simulink model "LFPrzeszkoda"  (R2024a)
settings: Solver=FixedStepDiscrete  StartTime=0.0  StopTime=2500  FixedStep=0.01  RelTol=1e-3
undefined symbols (not defined in the file): DiscIntNeverNeededParam, lineLength, mapForSim
libraries: mobileRoboticsTrainingLib x3, slpidlib x2
settings Model: PacingRate=50  Creator=KMPKM  LastModifiedBy=Pawel
settings RTWCC: GPUComputeCapability=3.5

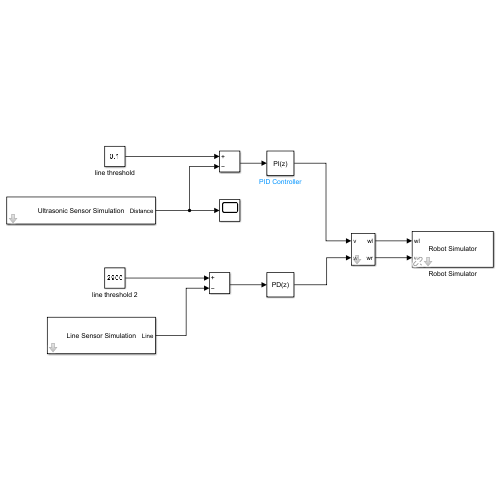
[thumbnail: Simulink's stored preview of the top-level diagram]
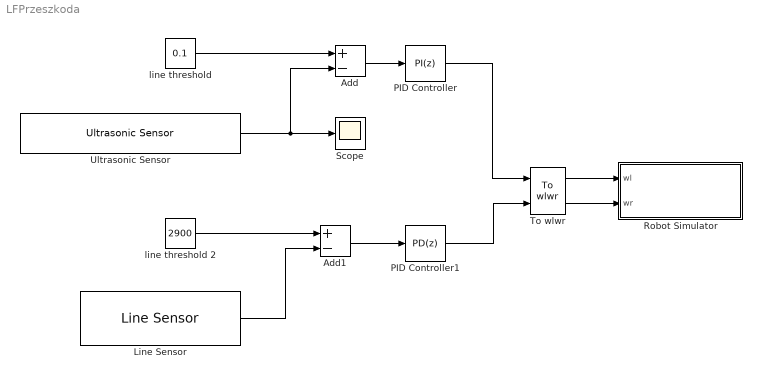
== system LFPrzeszkoda ==
  Add : Sum  Inputs=+-
  Add1 : Sum  Inputs=+-
  Line Sensor : mobileRoboticsTrainingLib/Line Sensor  mapVariable=mapForSim  envVal=2850  lineVal=2950  sensOff=[0.01 0]
      settings: SourceProductName=Mobile Robotics Training Library
  PID Controller : slpidlib/PID Controller  Controller=PI  Form=Parallel  TimeDomain=Discrete-time  UseExternalTs=off  SampleTime=-1  IntegratorMethod=Forward Euler  FilterMethod=Forward Euler  ControllerParametersSource=internal  P=1  I=0.001  UseKiTs=off  D=0.001  UseExternalDerivativeSource=off  N=100  UseFilter=on  TunerSelectOption=Transfer Function Based (PID Tuner App)  InitialConditionSource=internal  InitialConditionForIntegrator=0  InitialConditionForFilter=0  DifferentiatorICPrevScaledInput=0  ExternalReset=none  TrackingMode=off  Kt=1  LimitOutput=off  SatLimitsSource=internal  UpperSaturationLimit=inf  LowerSaturationLimit=-inf  LinearizeAsGain=on  AntiWindupMode=none  Kb=1  LimitIntegrator=off  UpperIntegratorSaturationLimit=inf  LowerIntegratorSaturationLimit=-inf  POutMin=[]  POutMax=[]  IOutMin=[]  IOutMax=[]  DOutMin=[]  DOutMax=[]  NOutMin=[]  NOutMax=[]  SumOutMin=[]  SumOutMax=[]  SaturationOutMin=[]  SaturationOutMax=[]  PParamMin=[]  PParamMax=[]  IParamMin=[]  IParamMax=[]  DParamMin=[]  DParamMax=[]  NParamMin=[]  NParamMax=[]  KbParamMin=[]  KbParamMax=[]  KtParamMin=[]  KtParamMax=[]  KbOutMin=[]  KbOutMax=[]  KtOutMin=[]  KtOutMax=[]  IntegratorOutMin=[]  IntegratorOutMax=[]  FilterOutMin=[]  FilterOutMax=[]  SumI1OutMin=[]  SumI1OutMax=[]  SumI2OutMin=[]  SumI2OutMax=[]  SumI3OutMin=[]  SumI3OutMax=[]  SumI4OutMin=[]  SumI4OutMax=[]  SumDOutMin=[]  SumDOutMax=[]  DifferentiatorOutMin=[]  DifferentiatorOutMax=[]  FilterDiffOutCoefMin=[]  FilterDiffOutCoefMax=[]  ReciprocalOutMin=[]  ReciprocalOutMax=[]  SumDenOutMin=[]  SumDenOutMax=[]  SumNumOutMin=[]  SumNumOutMax=[]  DivideOutMin=[]  DivideOutMax=[]  UdiffTsProdOutMin=[]  UdiffTsProdOutMax=[]  NTsProdOutMin=[]  NTsProdOutMax=[]  UintegralTsProdOutMin=[]  UintegralTsProdOutMax=[]  UngainTsProdOutMin=[]  UngainTsProdOutMax=[]  ClampingZeroOutDataTypeStr=Inherit: Inherit via back propagation  ClampingZeroOutMin=[]  ClampingZeroOutMax=[]  FilterDenConstantOutDataTypeStr=Inherit: Inherit via back propagation  FilterDenConstantOutMin=[]  FilterDenConstantOutMax=[]  PCopyOutDataTypeStr=Inherit: Inherit via back propagation  PCopyOutMin=[]  PCopyOutMax=[]  NCopyOutDataTypeStr=Inherit: Inherit via back propagation  NCopyOutMin=[]  NCopyOutMax=[]  IntegratorContinuousStateAttributes=''  IntegratorStateMustResolveToSignalObject=off  IntegratorRTWStateStorageClass=Auto  FilterContinuousStateAttributes=''  FilterStateMustResolveToSignalObject=off  FilterRTWStateStorageClass=Auto  ParallelPVariant=InternalParameters  IdealPVariant=Disabled  IVariant=InternalParameters  DVariant=Disabled  IntegratorVariant=Discrete  SatVariant=Disabled  AWVariant=Passthrough  PCopyVariant=Disabled  TRVariant=Disabled  FdbkBlocksVariant=Forward  IdealPFdbkVariant=Disabled  SatFdbkVariant=Disabled  DerivativeFilterVariant=Disabled  NVariant=Disabled  NCopyVariant=Disabled_SignalSpec  FilterICVariant=Disabled  IntegratorICVariant=InternalICs  ExternalResetVariant=Disabled  TRSumVariant=Passthrough  SumFdbkVariant=Disabled  SumVariant=Sum_PI  TsampFilterVariant=InternalTs  TsampNgainVariant=Passthrough  TsampIntegralVariant=Disabled_SignalSpec  ExternalSaturationOutDataTypeStr=Inherit: Same as second input  DerivativeSourceVariant=Disabled
  PID Controller1 : slpidlib/PID Controller  Controller=PD  Form=Parallel  TimeDomain=Discrete-time  UseExternalTs=off  SampleTime=-1  IntegratorMethod=Forward Euler  FilterMethod=Forward Euler  ControllerParametersSource=internal  P=0.01  I=1  UseKiTs=off  D=0.001  UseExternalDerivativeSource=off  N=100  UseFilter=on  TunerSelectOption=Transfer Function Based (PID Tuner App)  InitialConditionSource=internal  InitialConditionForIntegrator=0  InitialConditionForFilter=0  DifferentiatorICPrevScaledInput=0  ExternalReset=none  TrackingMode=off  Kt=1  LimitOutput=off  SatLimitsSource=internal  UpperSaturationLimit=inf  LowerSaturationLimit=-inf  LinearizeAsGain=on  AntiWindupMode=none  Kb=1  LimitIntegrator=off  UpperIntegratorSaturationLimit=inf  LowerIntegratorSaturationLimit=-inf  POutMin=[]  POutMax=[]  IOutMin=[]  IOutMax=[]  DOutMin=[]  DOutMax=[]  NOutMin=[]  NOutMax=[]  SumOutMin=[]  SumOutMax=[]  SaturationOutMin=[]  SaturationOutMax=[]  PParamMin=[]  PParamMax=[]  IParamMin=[]  IParamMax=[]  DParamMin=[]  DParamMax=[]  NParamMin=[]  NParamMax=[]  KbParamMin=[]  KbParamMax=[]  KtParamMin=[]  KtParamMax=[]  KbOutMin=[]  KbOutMax=[]  KtOutMin=[]  KtOutMax=[]  IntegratorOutMin=[]  IntegratorOutMax=[]  FilterOutMin=[]  FilterOutMax=[]  SumI1OutMin=[]  SumI1OutMax=[]  SumI2OutMin=[]  SumI2OutMax=[]  SumI3OutMin=[]  SumI3OutMax=[]  SumI4OutMin=[]  SumI4OutMax=[]  SumDOutMin=[]  SumDOutMax=[]  DifferentiatorOutMin=[]  DifferentiatorOutMax=[]  FilterDiffOutCoefMin=[]  FilterDiffOutCoefMax=[]  ReciprocalOutMin=[]  ReciprocalOutMax=[]  SumDenOutMin=[]  SumDenOutMax=[]  SumNumOutMin=[]  SumNumOutMax=[]  DivideOutMin=[]  DivideOutMax=[]  UdiffTsProdOutMin=[]  UdiffTsProdOutMax=[]  NTsProdOutMin=[]  NTsProdOutMax=[]  UintegralTsProdOutMin=[]  UintegralTsProdOutMax=[]  UngainTsProdOutMin=[]  UngainTsProdOutMax=[]  ClampingZeroOutDataTypeStr=Inherit: Inherit via back propagation  ClampingZeroOutMin=[]  ClampingZeroOutMax=[]  FilterDenConstantOutDataTypeStr=Inherit: Inherit via back propagation  FilterDenConstantOutMin=[]  FilterDenConstantOutMax=[]  PCopyOutDataTypeStr=Inherit: Inherit via back propagation  PCopyOutMin=[]  PCopyOutMax=[]  NCopyOutDataTypeStr=Inherit: Inherit via back propagation  NCopyOutMin=[]  NCopyOutMax=[]  IntegratorContinuousStateAttributes=''  IntegratorStateMustResolveToSignalObject=off  IntegratorRTWStateStorageClass=Auto  FilterContinuousStateAttributes=''  FilterStateMustResolveToSignalObject=off  FilterRTWStateStorageClass=Auto  ParallelPVariant=InternalParameters  IdealPVariant=Disabled  IVariant=Disabled  DVariant=InternalParameters  IntegratorVariant=Disabled  SatVariant=Disabled  AWVariant=Disabled  PCopyVariant=Disabled  TRVariant=Disabled  FdbkBlocksVariant=Forward  IdealPFdbkVariant=Disabled  SatFdbkVariant=Disabled  DerivativeFilterVariant=ForwardEulerFilter  NVariant=InternalParameters  NCopyVariant=Disabled  FilterICVariant=InternalICsFilter  IntegratorICVariant=Disabled  ExternalResetVariant=Disabled  TRSumVariant=Passthrough  SumFdbkVariant=Disabled  SumVariant=Sum_PD  TsampFilterVariant=InternalTs  TsampNgainVariant=Passthrough  TsampIntegralVariant=Disabled_SignalSpec  ExternalSaturationOutDataTypeStr=Inherit: Same as second input  DerivativeSourceVariant=ErrorSignal
  Robot Simulator : Subsystem  Priority=99  AncestorBlock=mobileRoboticsTrainingLib/Robot Simulator  mask(Robot Simulator){mapVar=[mapForSim], startX=54.1687, startY=51.2439, startTheta=0, axleLength=1, wheelR=0.5}
      mask prompts: mapVar "Map Variable"; startX "Start X (m)"; startY "Start Y (m)"; startTheta "Theta (deg)"; axleLength "Axle Length (m)"; wheelR "Wheel Radius (m)"
      mask help: Configure robot simulator to use custom simulation maps and simulate closed-loop mobile robotics systems along with appropriate sensor simulation blocks.
      mask init:
      | set_param(bdroot,'SolverType','Fixed-Step');
      | set_param(bdroot,'Solver','FixedStepDiscrete');
      | 
      | if (exist('Ts'))
      |     set_param(bdroot,'FixedStep','Ts');
      | else
      |     set_param(bdroot,'FixedStep','0.01');
      | end
      | 
      | h = findobj('Name','Robot Simulator');
      | if ~isempty(h)
      |     close (h);
      | end
      | setupRobotSim();
      mask Help: web('Robot Simulator.htm')
      mask DialogControl mapCont Prompt: Map Setup
      mask DialogControl initPosCont Prompt: Initial Position
      mask DialogControl setPos Prompt: Set position interactively
      mask DialogControl setPos Callback:
      | %% Set starting point
      | setStartingPoint();
      mask DialogControl initOrientation Prompt: Initial Orientation
      mask DialogControl robotCharCont Prompt: Robot Characteristics
      mask Display: disp('Robot Simulator')
  Scope : Scope
  To wlwr : mobileRoboticsTrainingLib/To wlwr  axleLength=0.1  wheelR=0.05
  Ultrasonic Sensor : mobileRoboticsTrainingLib/Ultrasonic Sensor  mapVar=mapForSim  maxSenRange=10  minSenRange=0.02  senRes=0.01  sensOff=[0 0]
      settings: SourceProductName=Mobile Robotics Training Library
  line threshold : Constant  Value=0.1
  line threshold 2 : Constant  Value=2900
  wires:
  To wlwr/1 -> Robot Simulator/1(wl)
  To wlwr/2 -> Robot Simulator/2(wr)
  line threshold/1 -> Add/1
  Ultrasonic Sensor/1 -> Add/2, Scope/1
  Add/1 -> PID Controller/1
  PID Controller/1 -> To wlwr/1
  line threshold 2/1 -> Add1/1
  Line Sensor/1 -> Add1/2
  Add1/1 -> PID Controller1/1
  PID Controller1/1 -> To wlwr/2

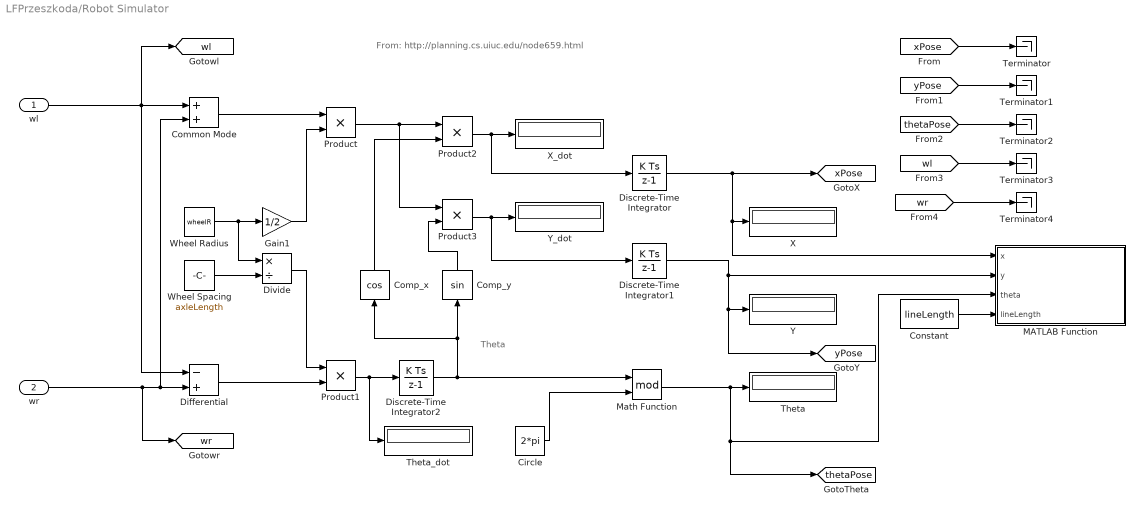
== system LFPrzeszkoda/Robot Simulator ==
  note: Theta
  note: From: http://planning.cs.uiuc.edu/node659.html
  wl : Inport
  wr : Inport  Port=2
  Circle : Constant  Value=2*pi
  Common Mode : Sum
  Comp_x : Trigonometry  Operator=cos
  Comp_y : Trigonometry
  Constant : Constant  Value=lineLength
  Differential : Sum  Inputs=-+
  Discrete-Time Integrator : DiscreteIntegrator  InitialCondition=startX  SampleTime=-1  ICPrevOutput=DiscIntNeverNeededParam  ICPrevScaledInput=DiscIntNeverNeededParam
  Discrete-Time Integrator1 : DiscreteIntegrator  InitialCondition=startY  SampleTime=-1  ICPrevOutput=DiscIntNeverNeededParam  ICPrevScaledInput=DiscIntNeverNeededParam
  Discrete-Time Integrator2 : DiscreteIntegrator  InitialCondition=startTheta*(pi/180)  SampleTime=-1  ICPrevOutput=DiscIntNeverNeededParam  ICPrevScaledInput=DiscIntNeverNeededParam
  Divide : Product  Inputs=*/
  Gain1 : Gain  Gain=1/2
  MATLAB Function : MATLAB Function  TreatAsAtomicUnit=on
  Math Function : Math  Operator=mod  SignedPower=on
  Product{,1..3} (4 alike) : Product  RndMeth=Zero
  Terminator{,1..4} (5 alike) : Terminator
  Theta : Display
  Theta_dot : Display
  Wheel Radius : Constant  Value=wheelR
  Wheel Spacing : Constant  Value=axleLength
  X : Display
  X_dot : Display
  Y : Display
  Y_dot : Display
  tag scope: thetaPose=global, wl=global, wr=global, xPose=global, yPose=global
  wires:
  [wr] -> Terminator4/1
  [wl] -> Terminator3/1
  Math Function/1 -> [thetaPose], MATLAB Function/3(theta), Theta/1
  Differential/1 -> Product1/2
  Comp_y/1 -> Product3/2
  Discrete-Time Integrator/1 -> [xPose], MATLAB Function/1(x), X/1
  Product3/1 -> Discrete-Time Integrator1/1, Y_dot/1
  Discrete-Time Integrator1/1 -> Y/1, [yPose], MATLAB Function/2(y)
  Divide/1 -> Product1/1
  wr/1 -> [wr], Common Mode/2, Differential/2
  Discrete-Time Integrator2/1 -> Math Function/1, Comp_x/1, Comp_y/1
  wl/1 -> [wl], Common Mode/1, Differential/1
  Comp_x/1 -> Product2/2
  Product1/1 -> Discrete-Time Integrator2/1, Theta_dot/1
  Wheel Radius/1 -> Divide/1, Gain1/1
  Wheel Spacing/1 -> Divide/2
  Product2/1 -> Discrete-Time Integrator/1, X_dot/1
  Gain1/1 -> Product/2
  Common Mode/1 -> Product/1
  Product/1 -> Product3/1, Product2/1
  Circle/1 -> Math Function/2
  Constant/1 -> MATLAB Function/4(lineLength)
  [xPose] -> Terminator/1
  [yPose] -> Terminator1/1
  [thetaPose] -> Terminator2/1

== matlab function LFPrzeszkoda/Robot Simulator/MATLAB Function ==
  data: x input; y input; theta input; lineLength input
function plotRobot(x,y,theta,lineLength)
% Get plot details
coder.extrinsic('evalin','plot')
ph1 = evalin('base','PlotHandle1');
ph2 = evalin('base','PlotHandle2');

% Find length orientation line
xp = [x x+lineLength*cos(theta)];
yp = [y y+lineLength*sin(theta)];

% Plot robot
set(ph1,'xdata',xp,'ydata',yp);
set(ph2,'xdata',x,'ydata',y);
drawnow('limitrate')
